simulink model "sen_acc_lib"  (R2020b)
settings: Solver=FixedStepDiscrete  StartTime=0.0  StopTime=20000  FixedStep=sen.imu_rate  RelTol=1e-3
undefined symbols (not defined in the file or in its folder): sen, sen_gyro_dyn_zeta, sen_gyro_lpf_wc
settings Model: Creator=jsint  LastModifiedBy=jsint

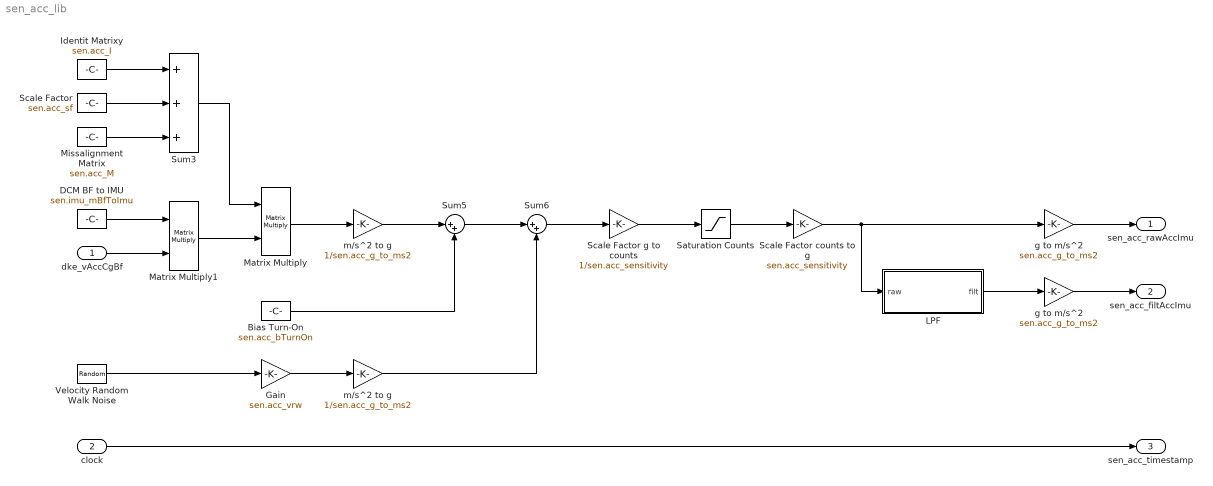
== system sen_acc_lib ==
  dke_vAccCgBf : Inport  OutDataTypeStr=double  Unit=rad/s  PortDimensions=[3,1]
  clock : Inport  Port=2  OutDataTypeStr=double  Unit=s  PortDimensions=[1,1]
  Bias Turn-On : Constant  Value=sen.acc_bTurnOn
  DCM BF to IMU : Constant  Value=sen.imu_mBfToImu
  Gain : Gain  Gain=sen.acc_vrw
  Identit Matrixy : Constant  Value=sen.acc_I
  LPF : Subsystem
  Matrix Multiply : Product  Multiplication=Matrix(*)
  Matrix Multiply1 : Product  Multiplication=Matrix(*)
  Missalignment Matrix : Constant  Value=sen.acc_M
  "Saturation Counts " : Saturate  UpperLimit=2^23  LowerLimit=-2^23
  Scale Factor : Constant  Value=sen.acc_sf
  Scale Factor counts to g : Gain  Gain=sen.acc_sensitivity
  Scale Factor g to counts : Gain  Gain=1/sen.acc_sensitivity
  Sum3 : Sum  Inputs=+++
  Sum5 : Sum  Inputs=|++
  Sum6 : Sum  Inputs=|++
  Velocity Random Walk Noise : RandomNumber  Seed=sen.acc_vrw_seed  SampleTime=sen.imu_rate
  g to m/s^2 : Gain  Gain=sen.acc_g_to_ms2
  "g to m/s^2 " : Gain  Gain=sen.acc_g_to_ms2
  m/s^2 to g : Gain  Gain=1/sen.acc_g_to_ms2
  "m/s^2 to g " : Gain  Gain=1/sen.acc_g_to_ms2
  sen_acc_rawAccImu : Outport  OutDataTypeStr=double  Unit=rad  PortDimensions=[3,1]
  sen_acc_filtAccImu : Outport  Port=2  OutDataTypeStr=double  Unit=rad  PortDimensions=[3,1]
  sen_acc_timestamp : Outport  Port=3  OutDataTypeStr=double  Unit=s  PortDimensions=[1,1]
  wires:
  Missalignment Matrix/1 -> Sum3/3
  Identit Matrixy/1 -> Sum3/1
  "Saturation Counts "/1 -> Scale Factor counts to g/1
  Gain/1 -> "m/s^2 to g "/1
  Velocity Random Walk Noise/1 -> Gain/1
  Sum5/1 -> Sum6/1
  Scale Factor g to counts/1 -> "Saturation Counts "/1
  Scale Factor/1 -> Sum3/2
  Sum3/1 -> Matrix Multiply/1
  Bias Turn-On/1 -> Sum5/2
  LPF/1(filt) -> "g to m/s^2 "/1
  clock/1 -> sen_acc_timestamp/1
  Matrix Multiply1/1 -> Matrix Multiply/2
  dke_vAccCgBf/1 -> Matrix Multiply1/2
  DCM BF to IMU/1 -> Matrix Multiply1/1
  Sum6/1 -> Scale Factor g to counts/1
  Scale Factor counts to g/1 -> g to m/s^2/1, LPF/1(raw)
  m/s^2 to g/1 -> Sum5/1
  Matrix Multiply/1 -> m/s^2 to g/1
  g to m/s^2/1 -> sen_acc_rawAccImu/1
  "g to m/s^2 "/1 -> sen_acc_filtAccImu/1
  "m/s^2 to g "/1 -> Sum6/2

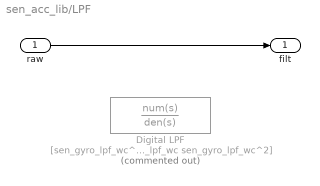
== system sen_acc_lib/LPF ==
  raw : Inport
  "Digital LPF " : TransferFcn  Commented=on  Numerator=[sen_gyro_lpf_wc^2]  Denominator=[1 2*sen_gyro_dyn_zeta*sen_gyro_lpf_wc sen_gyro_lpf_wc^2]
  filt : Outport
  wires:
  raw/1 -> filt/1
